simulink model "Digital_PWM_test"  (R2025b)
settings: Solver=VariableStepAuto  StartTime=0.0  StopTime=simStopTime  RelTol=1e-3
libraries: simulink x6
settings Model: Creator=Sneha Shree K  LastModifiedBy=Sneha Shree K

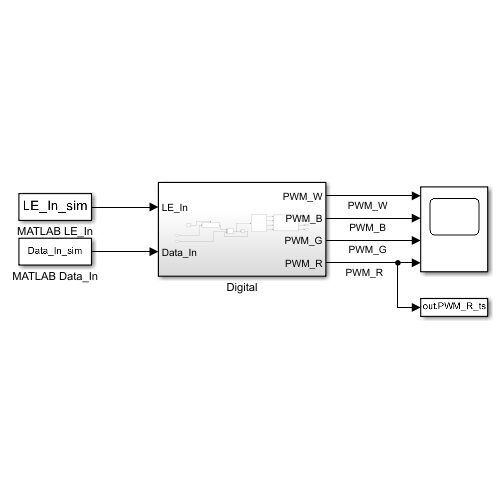
[thumbnail: Simulink's stored preview of the top-level diagram]
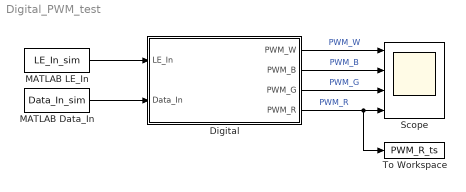
== system Digital_PWM_test ==
  Digital : Subsystem
  MATLAB Data_In : FromWorkspace  VariableName=Data_In_sim  Interpolate=off  OutputAfterFinalValue=Holding final value
  "MATLAB LE_In " : FromWorkspace  VariableName=LE_In_sim  Interpolate=off  OutputAfterFinalValue=Holding final value
  Scope : Scope  NumInputPorts=4
      settings: ActiveDisplayYMinimum=-0.41394567677319716  ActiveDisplayYMaximum=1.1355839256009383
  To Workspace : ToWorkspace  VariableName=PWM_R_ts  SaveFormat=Timeseries  SampleTime=-1
  wires:
  MATLAB Data_In/1 -> Digital/2(Data_In)
  "MATLAB LE_In "/1 -> Digital/1(LE_In)
  Digital/1(PWM_W) -> Scope/1  "PWM_W"
  Digital/2(PWM_B) -> Scope/2  "PWM_B"
  Digital/3(PWM_G) -> Scope/3  "PWM_G"
  Digital/4(PWM_R) -> To Workspace/1, Scope/4  "PWM_R"

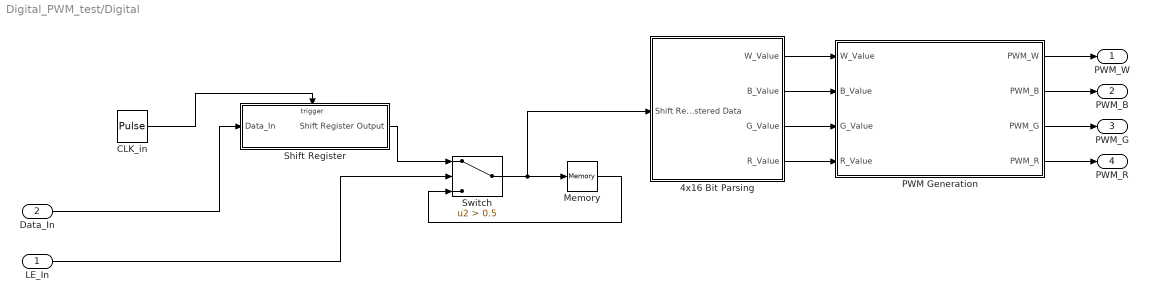
== system Digital_PWM_test/Digital ==
  LE_In : Inport
  Data_In : Inport  Port=2
  4x16 Bit Parsing : Subsystem
  CLK_in : DiscretePulseGenerator  PulseType=Time based  Period=1e-3  PulseWidth=50  PhaseDelay=0.5e-3
  Memory : Memory
  PWM Generation : Subsystem
  Shift Register : Subsystem  TreatAsAtomicUnit=on
  Switch : Switch  Criteria=u2 > Threshold  Threshold=0.5  SaturateOnIntegerOverflow=off  InputSameDT=off
  PWM_W : Outport
  PWM_B : Outport  Port=2
  PWM_G : Outport  Port=3
  PWM_R : Outport  Port=4
  wires:
  CLK_in/1 -> Shift Register/Trigger
  Data_In/1 -> Shift Register/1(Data_In)
  Switch/1 -> 4x16 Bit Parsing/1(Shift Registered Data), Memory/1
  Memory/1 -> Switch/3
  Shift Register/1(Shift Register Output) -> Switch/1
  LE_In/1 -> Switch/2
  4x16 Bit Parsing/1(W_Value) -> PWM Generation/1(W_Value)
  4x16 Bit Parsing/2(B_Value) -> PWM Generation/2(B_Value)
  4x16 Bit Parsing/3(G_Value) -> PWM Generation/3(G_Value)
  4x16 Bit Parsing/4(R_Value) -> PWM Generation/4(R_Value)
  PWM Generation/1(PWM_W) -> PWM_W/1
  PWM Generation/2(PWM_B) -> PWM_B/1
  PWM Generation/3(PWM_G) -> PWM_G/1
  PWM Generation/4(PWM_R) -> PWM_R/1

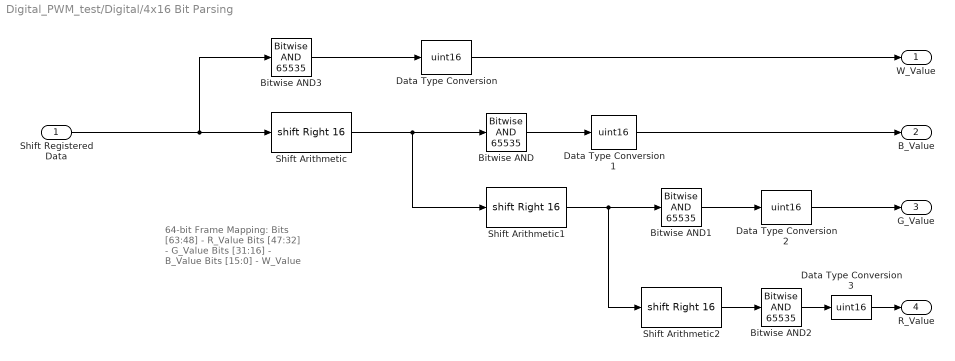
== system Digital_PWM_test/Digital/4x16 Bit Parsing ==
  note: 64-bit Frame Mapping:
      |
      | Bits [63:48] - R_Value
      | Bits [47:32] - G_Value
      | Bits [31:16] - B_Value
      | Bits [15:0] - W_Value
  Shift Registered Data : Inport  OutDataTypeStr=int64
  Bitwise AND{,1..3} (4 alike) : simulink/Logic and Bit Operations/Bitwise Operator  logicop=AND  UseBitMask=on  BitMask=65535  BitMaskRealWorld=Stored Integer
      settings: LibrarySourceBlock=|
      | simulink/Quick Insert/Logic and Bit
      | Operations/Bitwise AND
  Data Type Conversion{,1..3} (4 alike) : DataTypeConversion  OutDataTypeStr=uint16  SaturateOnIntegerOverflow=off  RndMeth=Floor
  Shift Arithmetic : ArithShift  BitShiftNumber=16  BitShiftDirection=Right
  Shift Arithmetic1 : ArithShift  BitShiftNumber=16  BitShiftDirection=Right
  Shift Arithmetic2 : ArithShift  BitShiftNumber=16  BitShiftDirection=Right
  W_Value : Outport
  B_Value : Outport  Port=2
  G_Value : Outport  Port=3
  R_Value : Outport  Port=4
  wires:
  Shift Arithmetic/1 -> Shift Arithmetic1/1, Bitwise AND/1
  Shift Registered Data/1 -> Shift Arithmetic/1, Bitwise AND3/1
  Shift Arithmetic1/1 -> Shift Arithmetic2/1, Bitwise AND1/1
  Shift Arithmetic2/1 -> Bitwise AND2/1
  Bitwise AND3/1 -> Data Type Conversion/1
  Bitwise AND/1 -> Data Type Conversion1/1
  Bitwise AND1/1 -> Data Type Conversion2/1
  Bitwise AND2/1 -> Data Type Conversion3/1
  Data Type Conversion/1 -> W_Value/1
  Data Type Conversion1/1 -> B_Value/1
  Data Type Conversion2/1 -> G_Value/1
  Data Type Conversion3/1 -> R_Value/1

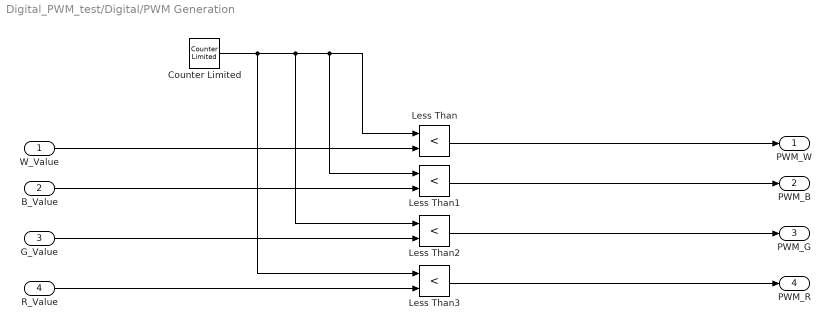
== system Digital_PWM_test/Digital/PWM Generation ==
  W_Value : Inport
  B_Value : Inport  Port=2
  G_Value : Inport  Port=3
  R_Value : Inport  Port=4
  Counter Limited : simulink/Sources/Counter Limited  uplimit=65535  tsamp=1e-6
  Less Than{,1..3} (4 alike) : RelationalOperator  Operator=<  OutDataTypeStr=boolean  RndMeth=Simplest  InputSameDT=off
  PWM_W : Outport
  PWM_B : Outport  Port=2
  PWM_G : Outport  Port=3
  PWM_R : Outport  Port=4
  wires:
  W_Value/1 -> Less Than/2
  Less Than/1 -> PWM_W/1
  Counter Limited/1 -> Less Than3/1, Less Than2/1, Less Than/1, Less Than1/1
  B_Value/1 -> Less Than1/2
  G_Value/1 -> Less Than2/2
  R_Value/1 -> Less Than3/2
  Less Than1/1 -> PWM_B/1
  Less Than2/1 -> PWM_G/1
  Less Than3/1 -> PWM_R/1

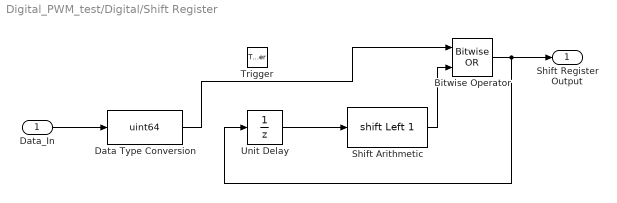
== system Digital_PWM_test/Digital/Shift Register ==
  Data_In : Inport
  Trigger : TriggerPort  VariantControl=(inherit)
  Bitwise Operator : simulink/Logic and Bit Operations/Bitwise Operator  logicop=OR  UseBitMask=off  NumInputPorts=2  BitMask=bin2dec('11011001')  BitMaskRealWorld=Stored Integer
  Data Type Conversion : DataTypeConversion  OutDataTypeStr=uint64  SaturateOnIntegerOverflow=off  RndMeth=Floor
  Shift Arithmetic : ArithShift  BitShiftNumber=1  BitShiftDirection=Left
  Unit Delay : UnitDelay  SampleTime=-1  HasFrameUpgradeWarning=on
  Shift Register Output : Outport  OutDataTypeStr=uint64
  wires:
  Data_In/1 -> Data Type Conversion/1
  Unit Delay/1 -> Shift Arithmetic/1
  Shift Arithmetic/1 -> Bitwise Operator/2
  Data Type Conversion/1 -> Bitwise Operator/1
  Bitwise Operator/1 -> Shift Register Output/1, Unit Delay/1
